simulink library "MulticopterModelLib"  (R2022a)
settings: Solver=VariableStepAuto  StartTime=0.0  StopTime=10.0  RelTol=1e-3
values from neighbouring files (symbols this model uses):
  ModelParam_envAltitude = -50    [Init.m]
  ModelParam_noiseGPSSampTime = 0.2    [Init.m]
undefined symbols (not defined in the file or in its folder): Earth, FaultParamAPI, SensorFault, WGS84
libraries: aerolibtransform2 x1
settings Model: Creator=dream  LastModifiedBy=Tujinhu
settings SolverCC: AlgebraicLoopSolver=TrustRegion
settings DataIOCC: ReturnWorkspaceOutputs=off
settings DebuggingCC: UnconnectedInputMsg=warning  UnconnectedOutputMsg=warning  UnconnectedLineMsg=warning  SFMachineParentedDataDiag=warning  ArithmeticOperatorsInVariantConditions=warning
settings SFSimCC: SimUseLocalCustomCode=off  CustomCodeUndefinedFunction=UseInterfaceOnly
settings RTWCC: RTWUseLocalCustomCode=off  DLArmComputeVersion=19.05

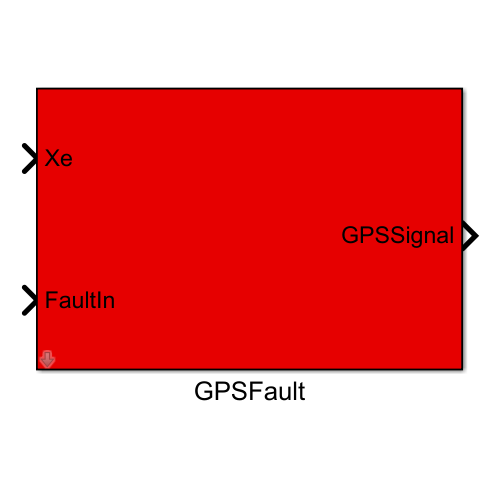
[thumbnail: Simulink's stored preview of the top-level diagram]
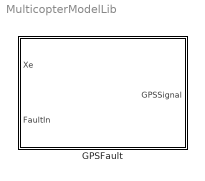
== system MulticopterModelLib ==
  GPSFault : Subsystem  mask{FaultParamStruct=SensorFault, ComParamVect=FaultParamAPI}
      mask prompts: FaultParamStruct "Fault Param Struct"; ComParamVect "Common Param Vect"
      mask DialogControl ParameterGroupVar Prompt: 参数

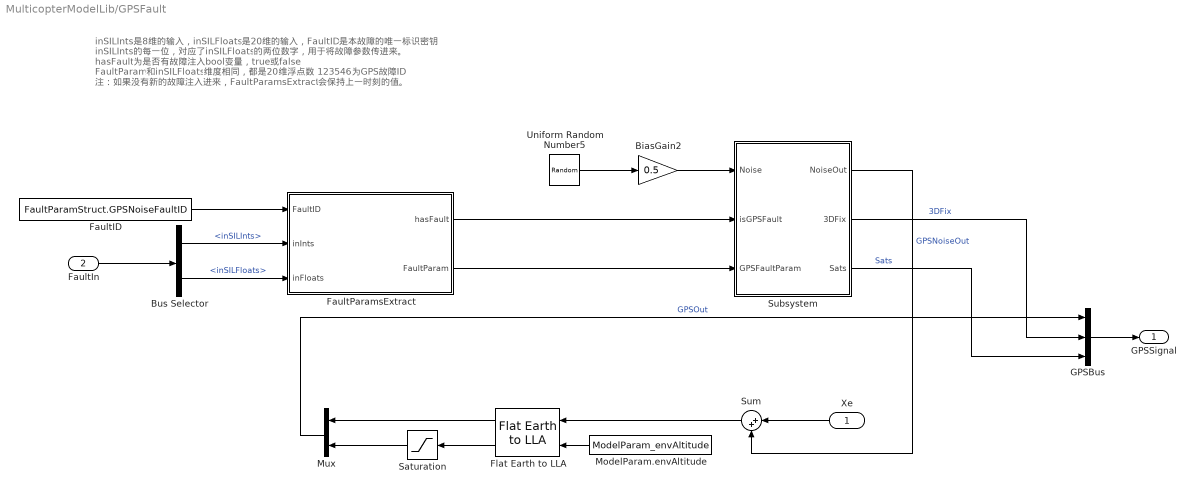
== system MulticopterModelLib/GPSFault ==
  note: inSILInts是8维的输入，inSILFloats是20维的输入，FaultID是本故障的唯一标识密钥
      | inSILInts的每一位，对应了inSILFloats的两位数字，用于将故障参数传进来。
      |
      | hasFault为是否有故障注入bool变量，true或false
      | FaultParam和inSILFloats维度相同，都是20维浮点数
      |
      | 123546为GPS故障ID
      |
      | 注：如果没有新的故障注入进来，FaultParamsExtract会保持上一时刻的值。
  Xe : Inport
  FaultIn : Inport  Port=2
  BiasGain2 : Gain  Gain=0.5
  Bus Selector : BusSelector  OutputSignals=inSILInts,inSILFloats
  FaultID : Constant  Value=FaultParamStruct.GPSNoiseFaultID  OutDataTypeStr=int32
  FaultParamsExtract : MATLAB Function  TreatAsAtomicUnit=on
  Flat Earth to LLA : aerolibtransform2/Flat Earth to LLA  units=Metric (MKS)  ptype=Earth (WGS84)  F=1/298.257223563  R=6378137  refPosPort=off  LL0=ModelParam_GPSLatLong  psi=0
  GPSBus : BusCreator  Inputs=3
  ModelParam.envAltitude : Constant  Value=ModelParam_envAltitude
  Mux : Mux  Inputs=2
  Saturation : Saturate  UpperLimit=100000  LowerLimit=0
  Subsystem : Subsystem
  Sum : Sum  Inputs=|++
  Uniform Random Number5 : UniformRandomNumber  Minimum=[-1,-1,-2]  Maximum=[1,1,2]  Seed=[1452,787,69]  SampleTime=ModelParam_noiseGPSSampTime
  GPSSignal : Outport
  wires:
  FaultParamsExtract/1(hasFault) -> Subsystem/2(isGPSFault)
  FaultParamsExtract/2(FaultParam) -> Subsystem/3(GPSFaultParam)
  Subsystem/3(Sats) -> GPSBus/3  "Sats"
  Saturation/1 -> Mux/2
  Flat Earth to LLA/2 -> Saturation/1
  Uniform Random Number5/1 -> BiasGain2/1
  FaultID/1 -> FaultParamsExtract/1(FaultID)
  BiasGain2/1 -> Subsystem/1(Noise)
  Bus Selector/1 -> FaultParamsExtract/2(inInts)  "<inSILInts>"
  FaultIn/1 -> Bus Selector/1
  Flat Earth to LLA/1 -> Mux/1
  Xe/1 -> Sum/1
  GPSBus/1 -> GPSSignal/1
  Subsystem/2(3DFix) -> GPSBus/2  "3DFix"
  ModelParam.envAltitude/1 -> Flat Earth to LLA/2
  Mux/1 -> GPSBus/1  "GPSOut"
  Subsystem/1(NoiseOut) -> Sum/2  "GPSNoiseOut"
  Bus Selector/2 -> FaultParamsExtract/3(inFloats)  "<inSILFloats>"
  Sum/1 -> Flat Earth to LLA/1

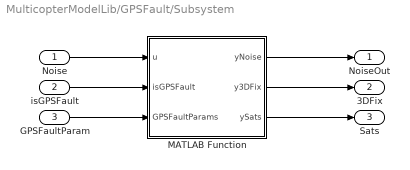
== system MulticopterModelLib/GPSFault/Subsystem ==
  Noise : Inport
  isGPSFault : Inport  Port=2
  GPSFaultParam : Inport  Port=3
  MATLAB Function : MATLAB Function  TreatAsAtomicUnit=on
  NoiseOut : Outport  VectorParamsAs1DForOutWhenUnconnected=off
  3DFix : Outport  Port=2  VectorParamsAs1DForOutWhenUnconnected=off
  Sats : Outport  Port=3  VectorParamsAs1DForOutWhenUnconnected=off
  wires:
  GPSFaultParam/1 -> MATLAB Function/3(GPSFaultParams)
  isGPSFault/1 -> MATLAB Function/2(isGPSFault)
  MATLAB Function/2(y3DFix) -> 3DFix/1
  MATLAB Function/3(ySats) -> Sats/1
  Noise/1 -> MATLAB Function/1(u)
  MATLAB Function/1(yNoise) -> NoiseOut/1

== matlab function MulticopterModelLib/GPSFault/Subsystem/MATLAB Function ==
  data: u input; yNoise output; isGPSFault input; GPSFaultParams input; y3DFix output; ySats output
function [yNoise,y3DFix,ySats] = fcn(u,isGPSFault,GPSFaultParams)

yNoise = u;
y3DFix = 3;
ySats = 10;

if isGPSFault
    yNoise = (GPSFaultParams(1))*u;
    y3DFix = GPSFaultParams(2);
    ySats = GPSFaultParams(3);
end

== matlab function MulticopterModelLib/GPSFault/FaultParamsExtract ==
  settings: updateMethod=DISCRETE
  data: FaultID input; inInts input; hasFault output; inFloats input; FaultParam output
function [hasFault, FaultParam] = fcn(FaultID,inInts,inFloats)
persistent hFault;
persistent fParam;

if isempty(hFault)
    hFault=false;
end
if isempty(fParam)
    fParam=zeros(20,1);
end

hFaultTmp=false;
fParamTmp=zeros(20,1);
j=1;
for i=1:8
    if inInts(i) == FaultID
        hFaultTmp=true;
        fParamTmp(2*j-1)=inFloats(2*i-1);
        fParamTmp(2*j)=inFloats(2*i);
        j=j+1;
    end
end
if hFaultTmp
    hFault=hFaultTmp;
    fParamTmp(17:20) = inFloats(17:20);
    fParam=fParamTmp;
end

hasFault=hFault;
FaultParam=fParam;
